simulink model "Group 2"  (R2024a)
settings: Solver=VariableStepAuto  StartTime=0.0  StopTime=1  RelTol=1e-3
undefined symbols (not defined in the file): Ion, Lithium
libraries: spsSeriesRLCBranchLib x6, spsDiodeLib x4, spsVoltageMeasurementLib x3, spsCurrentMeasurementLib x2, spsMosfetLib x2, simulink_need_slupdate x2, simulink x2, spsBatteryLib x1, spsPVArrayLib x1, sps_lib x1
settings Model: Creator=wchat  LastModifiedBy=wchat

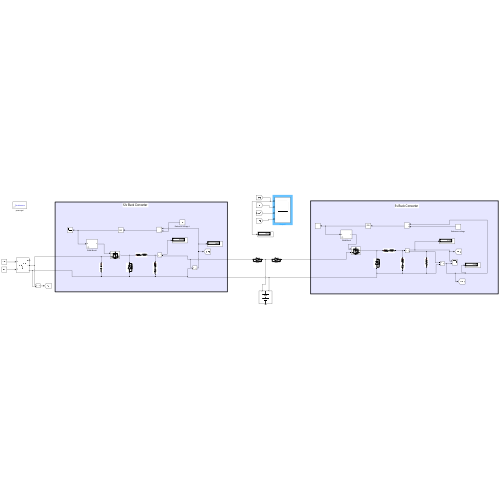
[thumbnail: Simulink's stored preview of the top-level diagram]
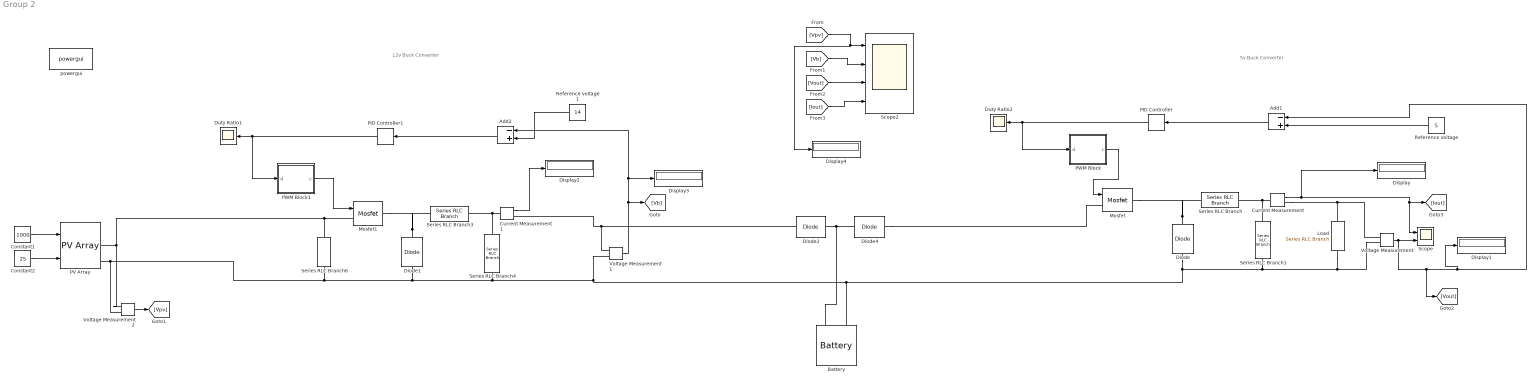
== system Group 2 ==
  note: 5v Buck Converter
  note: 12v Buck Converter
  Add1 : Sum  Inputs=-+
  Add2 : Sum  Inputs=-+
  Battery : spsBatteryLib/Battery  BatType=Lithium-Ion  ShowTempParam=off  ThermalPreset=no  ShowAgeParam=off  NomV=12  NomQ=100  SOC=40  Batt_Tr=30  PresetModel=off  MaxQ=100  MinV=9  FullV=14.4  Dis_rate=1  R=0.6  Normal_OP=90.4348  expZone="[12.9646      4.91304]"  current=[6.5 13 32.5]  Units=Time  Tci=20  NomT=20  T2=-30  MaxQ2=4.8  FullV2=7.1  Normal_OP2=5.655  expZone2="[6.58           1]"  Rca=0.6  ti=2000  Dp=0  Neq0=0  Tsim=1e6  Ta1=25  Qeol=5.4*0.9  Reol=0.013333*1.2  Char_age=[2.3478, 3]  Dis_age=[2.3478, 10]  N1=1500  N2=10500  N3=1000  N4=1400  Ta2=45  N5=950
  Constant1 : Constant  Value=1000
  Constant2 : Constant  Value=25
  Current Measurement : spsCurrentMeasurementLib/Current Measurement  PhasorSimulation=off  OutputType=Complex  PSBequivalent=0
  Current Measurement1 : spsCurrentMeasurementLib/Current Measurement  PhasorSimulation=off  OutputType=Complex  PSBequivalent=0
  Diode{,1..2,4} (4 alike) : spsDiodeLib/Diode  Ron=0.001  Lon=0  Vf=0.8  IC=0  UseSnubber=off  Rs=500  Cs=250e-9  Measurements=off
  Display{,1..4} (5 alike) : Display
  Duty Ratio1 : Scope
  Duty Ratio2 : Scope
  Load : spsSeriesRLCBranchLib/Series RLC Branch  LConnTagsString=__new0  RConnTagsString=__new0  BranchType=R  Resistance=1.67  Inductance=1e-3  SetiL0=off  InitialCurrent=0  Capacitance=1e-6  Setx0=off  InitialVoltage=0  Measurements=Branch voltage and current
  Mosfet : spsMosfetLib/Mosfet  Ron=0.1  Lon=0  Rd=0.01  Vfd=0  IC=0  Rs=1e5  Cs=inf  Measurements=off
  Mosfet1 : spsMosfetLib/Mosfet  Ron=0.1  Lon=0  Rd=0.01  Vfd=0  IC=0  Rs=1e5  Cs=inf  Measurements=off
  PID Controller : simulink_need_slupdate/PID Controller  P=0  I=1000  D=0
  PID Controller1 : simulink_need_slupdate/PID Controller  P=0  I=1000  D=0
  PV Array : spsPVArrayLib/PV Array  Npar=1  Nser=1  PlotType=array @ 1000 W/m2 & specified temperatures  S_vec="[ 1000  500  100 ]"  Temp_C_vec="[ 45 25  ]"  ModuleName=User-defined  PlotWhenSelected=off  Pm=59.94  Ncell=36  Voc=19  Isc=3.9  Vm=18  Im=3.33  beta_Voc_pc=-0.36099  alpha_Isc_pc=0.102  beta_Voc=-0.068588  alpha_Isc=0.003978  IL=3.9  I0=4.248e-10  nI=1.0008  Rsh=63.1583  Rs=0.0821  RobustModel=off  RobustCellTemperature=313.3991  BAL=on  Tc=1e-6  Tfilter=5e-5
  PWM Block : Subsystem  mask{fs=100e3}
      mask prompts: fs "Switching fFrequency"
  PWM Block1 : Subsystem  mask{fs=100e3}
      mask prompts: fs "Switching fFrequency"
  "Reference voltage " : Constant  Value=5
  Reference voltage 1 : Constant  Value=14
  Scope : Scope  NumInputPorts=2
  Scope2 : Scope  NumInputPorts=4
  Series RLC Branch : spsSeriesRLCBranchLib/Series RLC Branch  LConnTagsString=__new0  RConnTagsString=__new0  BranchType=RL  Resistance=80e-3  Inductance=34.5e-6  SetiL0=off  InitialCurrent=0  Capacitance=1e-6  Setx0=off  InitialVoltage=0  Measurements=None
  Series RLC Branch1 : spsSeriesRLCBranchLib/Series RLC Branch  LConnTagsString=__new0  RConnTagsString=__new0  BranchType=RC  Resistance=5e-3  Inductance=1e-3  SetiL0=off  InitialCurrent=0  Capacitance=22.5e-6  Setx0=off  InitialVoltage=0  Measurements=None
  Series RLC Branch3 : spsSeriesRLCBranchLib/Series RLC Branch  LConnTagsString=__new0  RConnTagsString=__new0  BranchType=RL  Resistance=80e-3  Inductance=85e-6  SetiL0=off  InitialCurrent=0  Capacitance=1e-6  Setx0=off  InitialVoltage=0  Measurements=None
  Series RLC Branch4 : spsSeriesRLCBranchLib/Series RLC Branch  LConnTagsString=__new0  RConnTagsString=__new0  BranchType=RC  Resistance=5e-3  Inductance=1e-3  SetiL0=off  InitialCurrent=0  Capacitance=3.75e-6  Setx0=off  InitialVoltage=0  Measurements=None
  Series RLC Branch6 : spsSeriesRLCBranchLib/Series RLC Branch  LConnTagsString=__new0  RConnTagsString=__new0  BranchType=C  Resistance=1.67  Inductance=1e-3  SetiL0=off  InitialCurrent=0  Capacitance=1e-6  Setx0=off  InitialVoltage=0  Measurements=None
  Voltage Measurement : spsVoltageMeasurementLib/Voltage Measurement  PhasorSimulation=off  OutputType=Complex  PSBequivalent=0
  Voltage Measurement1 : spsVoltageMeasurementLib/Voltage Measurement  PhasorSimulation=off  OutputType=Complex  PSBequivalent=0
  Voltage Measurement2 : spsVoltageMeasurementLib/Voltage Measurement  PhasorSimulation=off  OutputType=Complex  PSBequivalent=0
  powergui : sps_lib/powergui  Priority=1  SimulationMode=Continuous  SampleTime=1e-6  frequency=60  Iterations=50  frequencyindice=0  Pbase=100e6  ErrMax=1e-4  UnitsV=kV  UnitsW=MW  buscounter=0  FunctionMessages=off  echomessages=off  EnableUseOfTLC=off  CurrentSourceSwitches=on  DisableSnubberDevices=off  DisableRonSwitches=off  DisableVfSwitches=off  DisplayEquations=off  AutomaticDiscreteSolvers=off  SolverType=Tustin/Backward Euler (TBE)  Interpol=off  ExternalGateDelay=off  methode=off  Ts=0  x0status=blocks  SPID=off  SwTol=0  HookPort=off  NonlinearTolerance=1e-4  nMaxIteration=100  ContinueOnMaxIteration=off  RestoreLinks=warning  ResistiveCurrentMeasurement=off  Frange=[0:2:500]  Ylog=off  Xlog=on  ShowGrid=off  save=off  variable=ZData  structure=tpa14cfcc1_35b5_40eb_8b70_049b43167a68  ZoomFFT=off  StartTime=0.0  cycles=1  DisplayStyle=1  fundamental=60  FreqAxis=off  MaxFrequency=1000  frequencyindicesteady=1  RmsSteady=1  display=off
  wires:
  PID Controller/1 -> PWM Block/1(d), Duty Ratio2/1
  Current Measurement/1 -> Display/1, Scope/1, [Iout]
  Voltage Measurement/1 -> Scope/2, [Vout], Display1/1, Add1/1
  "Reference voltage "/1 -> Add1/2
  PWM Block/1(c) -> Mosfet/1
  Add1/1 -> PID Controller/1
  Reference voltage 1/1 -> Add2/2
  Add2/1 -> PID Controller1/1
  PWM Block1/1(c) -> Mosfet1/1
  PID Controller1/1 -> PWM Block1/1(d), Duty Ratio1/1
  Voltage Measurement1/1 -> [Vb], Add2/1, Display3/1
  Current Measurement1/1 -> Display2/1
  Constant2/1 -> PV Array/2
  Constant1/1 -> PV Array/1
  [Vpv] -> Display4/1, Scope2/1
  [Vb] -> Scope2/2
  [Vout] -> Scope2/3
  [Iout] -> Scope2/4
  Voltage Measurement2/1 -> [Vpv]
  connections:
  Current Measurement/RConn1 -- Voltage Measurement/LConn1 -- Load/LConn1
  Current Measurement/LConn1 -- Series RLC Branch1/LConn1 -- Series RLC Branch/RConn1
  Diode/RConn1 -- Mosfet/RConn1 -- Series RLC Branch/LConn1
  Diode4/RConn1 -- Mosfet/LConn1
  Current Measurement1/LConn1 -- Series RLC Branch4/LConn1 -- Series RLC Branch3/RConn1
  Load/RConn1 -- Voltage Measurement/LConn2 -- Series RLC Branch1/RConn1 -- Diode/LConn1 -- Battery/LConn2 -- Voltage Measurement1/LConn2 -- Diode1/LConn1 -- Series RLC Branch6/RConn1 -- Voltage Measurement2/LConn2 -- PV Array/RConn2 -- Series RLC Branch4/RConn1
  Diode1/RConn1 -- Mosfet1/RConn1 -- Series RLC Branch3/LConn1
  Diode2/LConn1 -- Voltage Measurement1/LConn1 -- Current Measurement1/RConn1
  Mosfet1/LConn1 -- Series RLC Branch6/LConn1 -- Voltage Measurement2/LConn1 -- PV Array/RConn1
  Diode2/RConn1 -- Battery/LConn1 -- Diode4/LConn1

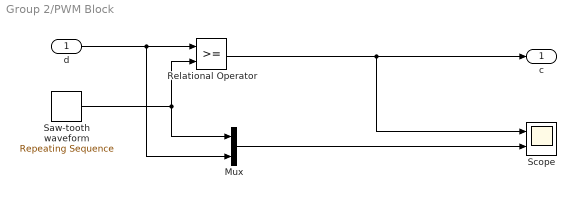
== system Group 2/PWM Block ==
  d : Inport
  Mux : Mux  Inputs=2
  Relational Operator : RelationalOperator  OutDataTypeStr=boolean  InputSameDT=off
  Saw-tooth waveform : simulink/Sources/Repeating Sequence  rep_seq_t=[0 1/fs]  rep_seq_y=[0 1]
  Scope : Scope  NumInputPorts=2
  c : Outport
  wires:
  d/1 -> Mux/2, Relational Operator/1
  Saw-tooth waveform/1 -> Mux/1, Relational Operator/2
  Relational Operator/1 -> c/1, Scope/1
  Mux/1 -> Scope/2

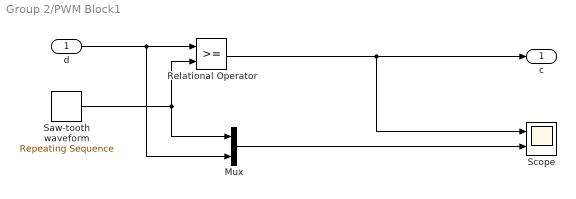
== system Group 2/PWM Block1 ==
  d : Inport
  Mux : Mux  Inputs=2
  Relational Operator : RelationalOperator  OutDataTypeStr=boolean  InputSameDT=off
  Saw-tooth waveform : simulink/Sources/Repeating Sequence  rep_seq_t=[0 1/fs]  rep_seq_y=[0 1]
  Scope : Scope  NumInputPorts=2
  c : Outport
  wires:
  d/1 -> Mux/2, Relational Operator/1
  Saw-tooth waveform/1 -> Mux/1, Relational Operator/2
  Relational Operator/1 -> c/1, Scope/1
  Mux/1 -> Scope/2
